simulink library "acc"  (Simulink 8.1)
settings: Solver=ode1  StartTime=0.0  StopTime=Inf  FixedStep=0.001  RelTol=1e-3
PostLoadFcn:
  | , if any(exist('dsrtsu_mdlpostloadfcn', 'file') == [2, 3, 6]), try dsrtsu_mdlpostloadfcn('Execute', bdroot); catch fprintf('Error in PostLoadFcn (dsrtsu_mdlpostloadfcn) for model "%s":\n %s\n', bdroot, lasterr); end, end,
undefined symbols (not defined in the file or in its folder): FALSE, KACC_DefStandstillClearance_m
libraries: cac x1, scc x1
settings Model: DSRTSU_INTERNAL_RTI_VER=450  DSRTSU_INTERNAL_RTI_TYPE=rti1401  RTICANMMDATA=struct('GeneralSetupData',struct('modelroot','D:\ELN150201_TAIWAN\trunk\AdasDragon\software\sw_development\arch\app\acc','generalsettings',struct('filesettings',struct('destfolder',struct('Name','RTICANMM_FILES','Check',1),'buildfolder',struct('Name','.','Check',1),'AbsDestfolder',struct('Name','D:\ELN150201_TAIWAN\trunk\AdasDragon\software\sw_development\arch\app\acc\RTICANMM_FILES'),'AbsBuildfolder',struct('Name','D:\ELN150201_TAIWAN\trunk\AdasDragon\software\sw_development\arch\app\acc'))),'options',struct('addpaths',1,'rmpaths',1,'addtrcexclusion',logical(1),'cannavigator',struct('checkmonitoring',0),'show_usrtrc',0,'use_usrtrc',0),'advanced',struct('options',[1 1 1 1 1 1 1 1 1 1 1 1 1 1 1 1 1 1 1 1 1 1 1 1 1 1 1 1 1 1 1 1 1 1 1 1 1 1 1 1 1 1 1 1 1 1 1 1 1 1 1 1 1 1 1 1 1 1 1 1 1 1 1 1 1 1 1 1 1 1 1 1 1 1 1 1 1 1 1 1 1 1 1 1 1 1 1 1 1 1 1 1 1 1 1 1 1 1 1 1]),'MPSetup',{{}},'modelname','acc','block','acc'))  DSRTSU_INTERNAL_RTIFPGA=40  Creator=AT015411  LastModifiedBy=AT015555

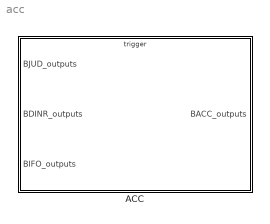
== system acc ==
  ACC : Subsystem

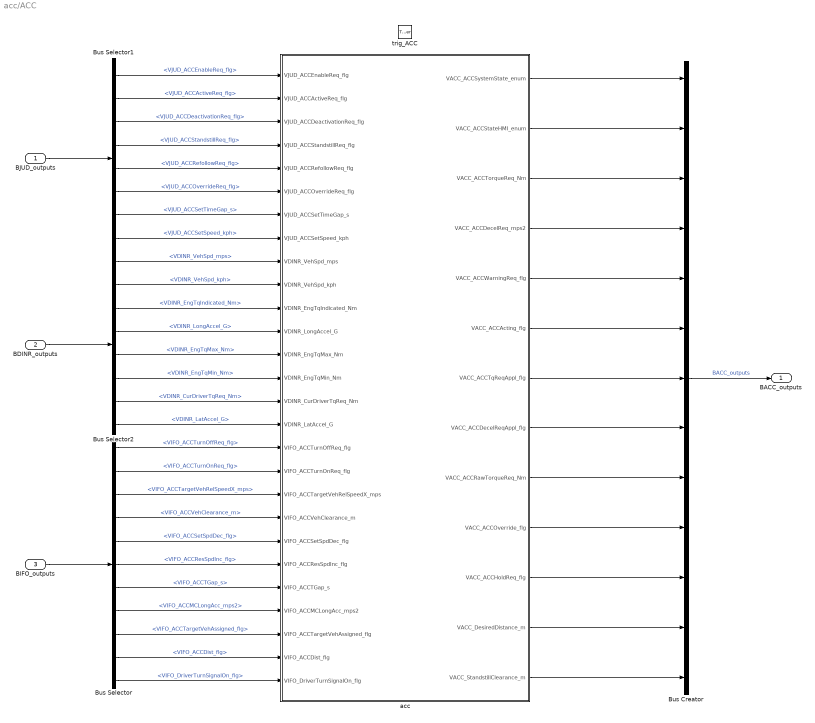
== system acc/ACC ==
  BJUD_outputs : Inport  OutDataTypeStr=Bus: BJUD_outputs
  BDINR_outputs : Inport  Port=2  OutDataTypeStr=Bus: BDINR_outputs
  BIFO_outputs : Inport  Port=3  OutDataTypeStr=Bus: BIFO_outputs
  trig_ACC : TriggerPort  TriggerType=function-call
      settings: AttributesFormatString=State = %<StatesWhenEnabling>
  Bus Creator : BusCreator  Inputs=13  OutDataTypeStr=Bus: BACC_outputs
  Bus Selector : BusSelector  OutputSignals=VIFO_ACCTurnOffReq_flg,VIFO_ACCTurnOnReq_flg,VIFO_ACCTargetVehRelSpeedX_mps,VIFO_ACCVehClearance_m,VIFO_ACCSetSpdDec_flg,VIFO_ACCResSpdInc_flg,VIFO_ACCTGap_s,VIFO_ACCMCLongAcc_mps2,VIFO_ACCTargetVehAssigned_flg,VIFO_ACCDist_flg,VIFO_DriverTurnSignalOn_flg
  Bus Selector1 : BusSelector  OutputSignals=VJUD_ACCEnableReq_flg,VJUD_ACCActiveReq_flg,VJUD_ACCDeactivationReq_flg,VJUD_ACCStandstillReq_flg,VJUD_ACCRefollowReq_flg,VJUD_ACCOverrideReq_flg,VJUD_ACCSetTimeGap_s,VJUD_ACCSetSpeed_kph
  Bus Selector2 : BusSelector  OutputSignals=VDINR_VehSpd_mps,VDINR_VehSpd_kph,VDINR_EngTqIndicated_Nm,VDINR_LongAccel_G,VDINR_EngTqMax_Nm,VDINR_EngTqMin_Nm,VDINR_CurDriverTqReq_Nm,VDINR_LatAccel_G
  acc : Subsystem
  BACC_outputs : Outport  OutDataTypeStr=Bus: BACC_outputs
  wires:
  Bus Selector/11 -> acc/27(VIFO_DriverTurnSignalOn_flg)  "<VIFO_DriverTurnSignalOn_flg>"
  Bus Selector2/3 -> acc/11(VDINR_EngTqIndicated_Nm)  "<VDINR_EngTqIndicated_Nm>"
  Bus Selector/5 -> acc/21(VIFO_ACCSetSpdDec_flg)  "<VIFO_ACCSetSpdDec_flg>"
  Bus Selector/6 -> acc/22(VIFO_ACCResSpdInc_flg)  "<VIFO_ACCResSpdInc_flg>"
  Bus Selector/7 -> acc/23(VIFO_ACCTGap_s)  "<VIFO_ACCTGap_s>"
  Bus Selector/8 -> acc/24(VIFO_ACCMCLongAcc_mps2)  "<VIFO_ACCMCLongAcc_mps2>"
  Bus Selector/9 -> acc/25(VIFO_ACCTargetVehAssigned_flg)  "<VIFO_ACCTargetVehAssigned_flg>"
  BIFO_outputs/1 -> Bus Selector/1
  BJUD_outputs/1 -> Bus Selector1/1
  Bus Creator/1 -> BACC_outputs/1  "BACC_outputs"
  BDINR_outputs/1 -> Bus Selector2/1
  Bus Selector1/1 -> acc/1(VJUD_ACCEnableReq_flg)  "<VJUD_ACCEnableReq_flg>"
  Bus Selector1/2 -> acc/2(VJUD_ACCActiveReq_flg)  "<VJUD_ACCActiveReq_flg>"
  Bus Selector1/4 -> acc/4(VJUD_ACCStandstillReq_flg)  "<VJUD_ACCStandstillReq_flg>"
  Bus Selector1/5 -> acc/5(VJUD_ACCRefollowReq_flg)  "<VJUD_ACCRefollowReq_flg>"
  Bus Selector1/3 -> acc/3(VJUD_ACCDeactivationReq_flg)  "<VJUD_ACCDeactivationReq_flg>"
  Bus Selector1/6 -> acc/6(VJUD_ACCOverrideReq_flg)  "<VJUD_ACCOverrideReq_flg>"
  Bus Selector2/4 -> acc/12(VDINR_LongAccel_G)  "<VDINR_LongAccel_G>"
  Bus Selector2/5 -> acc/13(VDINR_EngTqMax_Nm)  "<VDINR_EngTqMax_Nm>"
  Bus Selector2/6 -> acc/14(VDINR_EngTqMin_Nm)  "<VDINR_EngTqMin_Nm>"
  Bus Selector/2 -> acc/18(VIFO_ACCTurnOnReq_flg)  "<VIFO_ACCTurnOnReq_flg>"
  Bus Selector/1 -> acc/17(VIFO_ACCTurnOffReq_flg)  "<VIFO_ACCTurnOffReq_flg>"
  Bus Selector2/7 -> acc/15(VDINR_CurDriverTqReq_Nm)  "<VDINR_CurDriverTqReq_Nm>"
  Bus Selector2/8 -> acc/16(VDINR_LatAccel_G)  "<VDINR_LatAccel_G>"
  Bus Selector/3 -> acc/19(VIFO_ACCTargetVehRelSpeedX_mps)  "<VIFO_ACCTargetVehRelSpeedX_mps>"
  Bus Selector/4 -> acc/20(VIFO_ACCVehClearance_m)  "<VIFO_ACCVehClearance_m>"
  Bus Selector1/7 -> acc/7(VJUD_ACCSetTimeGap_s)  "<VJUD_ACCSetTimeGap_s>"
  Bus Selector1/8 -> acc/8(VJUD_ACCSetSpeed_kph)  "<VJUD_ACCSetSpeed_kph>"
  Bus Selector/10 -> acc/26(VIFO_ACCDist_flg)  "<VIFO_ACCDist_flg>"
  Bus Selector2/2 -> acc/10(VDINR_VehSpd_kph)  "<VDINR_VehSpd_kph>"
  acc/1(VACC_ACCSystemState_enum) -> Bus Creator/1
  acc/2(VACC_ACCStateHMI_enum) -> Bus Creator/2
  acc/3(VACC_ACCTorqueReq_Nm) -> Bus Creator/3
  acc/4(VACC_ACCDecelReq_mps2) -> Bus Creator/4
  acc/5(VACC_ACCWarningReq_flg) -> Bus Creator/5
  acc/6(VACC_ACCActing_flg) -> Bus Creator/6
  acc/7(VACC_ACCTqReqAppl_flg) -> Bus Creator/7
  acc/8(VACC_ACCDecelReqAppl_flg) -> Bus Creator/8
  acc/9(VACC_ACCRawTorqueReq_Nm) -> Bus Creator/9
  acc/10(VACC_ACCOverride_flg) -> Bus Creator/10
  acc/11(VACC_ACCHoldReq_flg) -> Bus Creator/11
  acc/12(VACC_DesiredDistance_m) -> Bus Creator/12
  Bus Selector2/1 -> acc/9(VDINR_VehSpd_mps)  "<VDINR_VehSpd_mps>"
  acc/13(VACC_StandstillClearance_m) -> Bus Creator/13

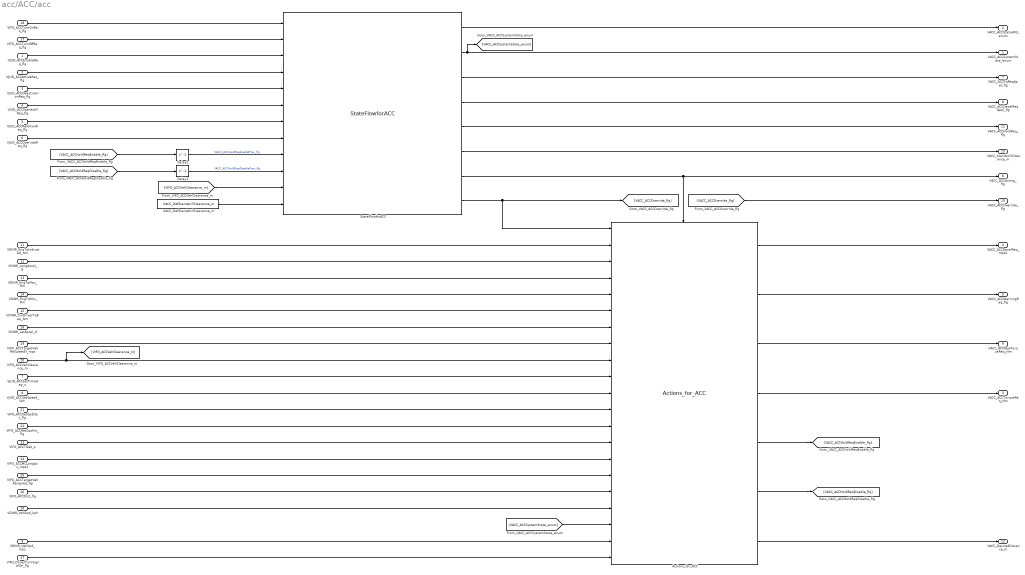
== system acc/ACC/acc ==
  VJUD_ACCEnableReq_flg : Inport
  VJUD_ACCActiveReq_flg : Inport  Port=2
  VJUD_ACCDeactivationReq_flg : Inport  Port=3
  VJUD_ACCStandstillReq_flg : Inport  Port=4
  VJUD_ACCRefollowReq_flg : Inport  Port=5
  VJUD_ACCOverrideReq_flg : Inport  Port=6
  VJUD_ACCSetTimeGap_s : Inport  Port=7
  VJUD_ACCSetSpeed_kph : Inport  Port=8
  VDINR_VehSpd_mps : Inport  Port=9
  VDINR_VehSpd_kph : Inport  Port=10
  VDINR_EngTqIndicated_Nm : Inport  Port=11
  VDINR_LongAccel_G : Inport  Port=12
  VDINR_EngTqMax_Nm : Inport  Port=13
  VDINR_EngTqMin_Nm : Inport  Port=14
  VDINR_CurDriverTqReq_Nm : Inport  Port=15
  VDINR_LatAccel_G : Inport  Port=16
  VIFO_ACCTurnOffReq_flg : Inport  Port=17
  VIFO_ACCTurnOnReq_flg : Inport  Port=18
  VIFO_ACCTargetVehRelSpeedX_mps : Inport  Port=19
  VIFO_ACCVehClearance_m : Inport  Port=20
  VIFO_ACCSetSpdDec_flg : Inport  Port=21
  VIFO_ACCResSpdInc_flg : Inport  Port=22
  VIFO_ACCTGap_s : Inport  Port=23
  VIFO_ACCMCLongAcc_mps2 : Inport  Port=24
  VIFO_ACCTargetVehAssigned_flg : Inport  Port=25
  VIFO_ACCDist_flg : Inport  Port=26
  VIFO_DriverTurnSignalOn_flg : Inport  Port=27
  Actions_for_ACC : cac/Actions_for_ACC
  Delay1 : Delay  DelayLength=1  InitialCondition=0
  Delay2 : Delay  DelayLength=1  InitialCondition=0
  KACC_DefStandstillClearance_m : Constant  Value=KACC_DefStandstillClearance_m
  StateFlowforACC : scc/StateFlowforACC
  VACC_ACCSystemState_enum : Outport
  VACC_ACCStateHMI_enum : Outport  Port=2
  VACC_ACCTorqueReq_Nm : Outport  Port=3
  VACC_ACCDecelReq_mps2 : Outport  Port=4
  VACC_ACCWarningReq_flg : Outport  Port=5
  VACC_ACCActing_flg : Outport  Port=6
  VACC_ACCTqReqAppl_flg : Outport  Port=7
  VACC_ACCDecelReqAppl_flg : Outport  Port=8
  VACC_ACCRawTorqueReq_Nm : Outport  Port=9
  VACC_ACCOverride_flg : Outport  Port=10
  VACC_ACCHoldReq_flg : Outport  Port=11
  VACC_DesiredDistance_m : Outport  Port=12  OutputWhenDisabled=reset  InitialOutput=FALSE
  VACC_StandstillClearance_m : Outport  Port=13
  wires:
  VDINR_EngTqIndicated_Nm/1 -> Actions_for_ACC/2
  VIFO_ACCResSpdInc_flg/1 -> Actions_for_ACC/13
  VIFO_ACCSetSpdDec_flg/1 -> Actions_for_ACC/12
  Actions_for_ACC/1 -> VACC_ACCDecelReq_mps2/1
  VIFO_ACCTurnOnReq_flg/1 -> StateFlowforACC/1
  VIFO_ACCTurnOffReq_flg/1 -> StateFlowforACC/2
  VJUD_ACCActiveReq_flg/1 -> StateFlowforACC/4
  VJUD_ACCDeactivationReq_flg/1 -> StateFlowforACC/5
  VJUD_ACCStandstillReq_flg/1 -> StateFlowforACC/6
  VJUD_ACCRefollowReq_flg/1 -> StateFlowforACC/7
  VJUD_ACCOverrideReq_flg/1 -> StateFlowforACC/8
  VDINR_CurDriverTqReq_Nm/1 -> Actions_for_ACC/6
  VDINR_EngTqMin_Nm/1 -> Actions_for_ACC/5
  VDINR_EngTqMax_Nm/1 -> Actions_for_ACC/4
  VDINR_LongAccel_G/1 -> Actions_for_ACC/3
  StateFlowforACC/1 -> VACC_ACCStateHMI_enum/1
  StateFlowforACC/2 -> VACC_ACCSystemState_enum/1, [VACC_ACCSystemState_enum]
  StateFlowforACC/4 -> VACC_ACCDecelReqAppl_flg/1
  StateFlowforACC/3 -> VACC_ACCTqReqAppl_flg/1
  VDINR_LatAccel_G/1 -> Actions_for_ACC/7
  StateFlowforACC/8 -> [VACC_ACCOverride_flg], Actions_for_ACC/1
  VIFO_ACCVehClearance_m/1 -> Actions_for_ACC/9, [VIFO_ACCVehClearance_m]
  VIFO_ACCTargetVehRelSpeedX_mps/1 -> Actions_for_ACC/8
  VJUD_ACCSetTimeGap_s/1 -> Actions_for_ACC/10
  VJUD_ACCSetSpeed_kph/1 -> Actions_for_ACC/11
  VIFO_ACCTargetVehAssigned_flg/1 -> Actions_for_ACC/16
  VIFO_ACCTGap_s/1 -> Actions_for_ACC/14
  VIFO_ACCMCLongAcc_mps2/1 -> Actions_for_ACC/15
  StateFlowforACC/7 -> Actions_for_ACC/Enable, VACC_ACCActing_flg/1
  VIFO_ACCDist_flg/1 -> Actions_for_ACC/17
  [VACC_ACCOverride_flg] -> VACC_ACCOverride_flg/1
  Actions_for_ACC/2 -> VACC_ACCWarningReq_flg/1
  Actions_for_ACC/3 -> VACC_ACCRawTorqueReq_Nm/1
  Actions_for_ACC/4 -> VACC_ACCTorqueReq_Nm/1
  Actions_for_ACC/5 -> [VACC_ACCHoldReqEnable_flg]
  Actions_for_ACC/6 -> [VACC_ACCHoldReqDisable_flg]
  VDINR_VehSpd_kph/1 -> Actions_for_ACC/18
  [VACC_ACCHoldReqEnable_flg] -> Delay2/1
  [VACC_ACCHoldReqDisable_flg] -> Delay1/1
  VJUD_ACCEnableReq_flg/1 -> StateFlowforACC/3
  Delay1/1 -> StateFlowforACC/10  "VACC_ACCHoldReqDisablePrev_flg"
  Delay2/1 -> StateFlowforACC/9  "VACC_ACCHoldReqEnablePrev_flg"
  StateFlowforACC/5 -> VACC_ACCHoldReq_flg/1
  Actions_for_ACC/7 -> VACC_DesiredDistance_m/1
  [VACC_ACCSystemState_enum] -> Actions_for_ACC/19
  VDINR_VehSpd_mps/1 -> Actions_for_ACC/20
  StateFlowforACC/6 -> VACC_StandstillClearance_m/1
  [VIFO_ACCVehClearance_m] -> StateFlowforACC/11
  KACC_DefStandstillClearance_m/1 -> StateFlowforACC/12
  VIFO_DriverTurnSignalOn_flg/1 -> Actions_for_ACC/21
